simulink model "recursive_variable_window_size_alg_RL"  (R2019b)
settings: Solver=ode45  StartTime=0.0  StopTime=0.6  MaxStep=1e-4  RelTol=1e-4  AbsTol=1e-6
values from neighbouring files (symbols this model uses):
  den = [1]    [dab1.m]
  dx = 0    [dab1.m]
  num = [1]    [dab1.m]
libraries: elements x2, simulink x2, simulink_extras x1
settings Model: ExtModeTrigMode=oneshot  ExtModeArmWhenConnect=off  Creator=PC  LastModifiedBy=bae_rashid
settings SolverCC: AutoScaleAbsTol=off
settings DataIOCC: SaveFormat=Array  ReturnWorkspaceOutputs=off
settings OptimizationCC: BlockReduction=off  BooleanDataType=off  LifeSpan=inf
settings DebuggingCC: SaveWithParameterizedLinksMsg=none  UnderspecifiedInitializationDetection=Classic  MergeDetectMultiDrivingBlocksExec=none  SignalResolutionControl=TryResolveAllWithWarning  MultiTaskDSMMsg=warning  MultiTaskCondExecSysMsg=none  SFUnexpectedBacktrackingDiag=warning  SFNoUnconditionalDefaultTransitionDiag=warning  SFExecutionAtInitializationDiag=none  ArithmeticOperatorsInVariantConditions=warning
settings HardwareCC: ProdBitPerPointer=32  ProdBitPerSizeT=32  ProdBitPerPtrDiffT=32  ProdLargestAtomicFloat=None  ProdIntDivRoundTo=Undefined  ProdEndianess=Unspecified  ProdWordSize=32  ProdHWDeviceType=32-bit Generic  TargetUnknown=on
settings ModelReferenceCC: PropagateSignalLabelsOutOfModel=off
settings SFSimCC: SimUseLocalCustomCode=off  CustomCodeUndefinedFunction=UseInterfaceOnly
settings RTWCC: TemplateMakefile=grt_vc.tmf  RTWUseLocalCustomCode=off
settings CodeAppCC: StateflowObjectComments=on
settings GRTTargetCC: TargetLangStandard=C89/C90 (ANSI)  GeneratePreprocessorConditionals=Disable all  CombineOutputUpdateFcns=off  GRTInterface=on
settings ConfigComp: CovMetricSettings=dw  CovHtmlReporting=on  CovSaveCumulativeToWorkspaceVar=on  CovSaveSingleToWorkspaceVar=on  CovExternalEMLEnable=off

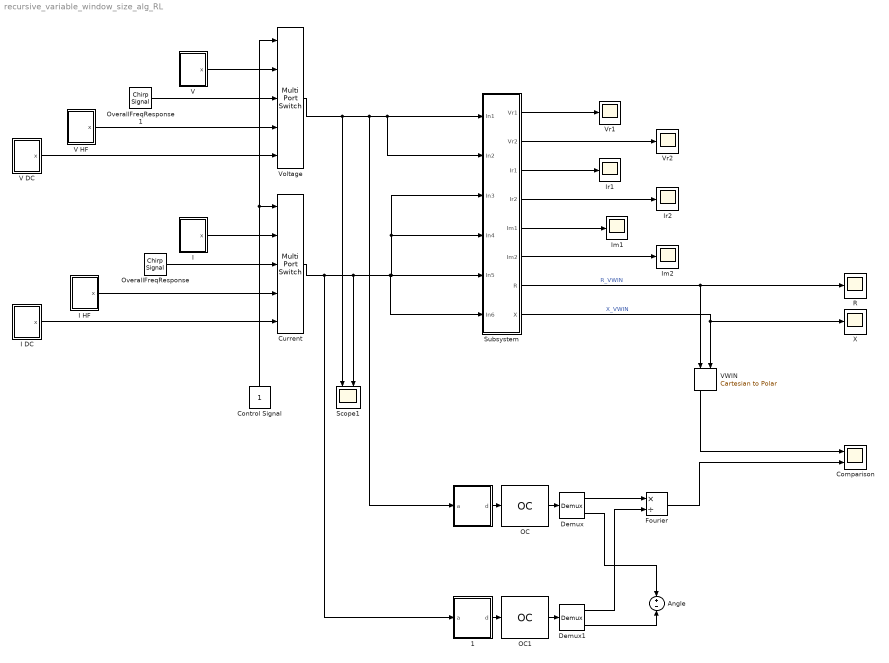
== system recursive_variable_window_size_alg_RL ==
  "  " : Subsystem  mask(Data Adquisition Board){filter=on, approx=Butterworth, order=3, numerator=[], denominator=[], freq=180, resdis=on, vertres=8, xmax=100, winsize=60, G=1.0, fs=60*60}
      mask prompts: filter "Disable Analog Filter"; approx "Filter approximation"; numerator "Free expression filter: numerator(descending order of s)"; denominator "Free expression filter: denominator:"; freq "Cut-off frequency"; resdis "Disable Vertical Resolution"; vertres "Vertical Resolution: No. of bits"; xmax "Vertical Resolution: signal range"; winsize "Window size"; G "Gain"; fs "Sampling frequency"
      mask help: Takes the instantaneous value of the input signal and convert it to the data window of samples.
      mask init:
      | dab1
      mask TypeOptions approx: Bessel | Tschebyscheff | Butterworth | free expression
      mask TypeOptions order: 2 | 3 | 4
      mask TypeOptions vertres: 8 | 12 | 16
      mask Display: disp('DAB')
  "  1" : Subsystem  mask(Data Adquisition Board){filter=on, approx=Butterworth, order=3, numerator=[], denominator=[], freq=180, resdis=on, vertres=8, xmax=100, winsize=60, G=1.0, fs=60*60}
      mask prompts: filter "Disable Analog Filter"; approx "Filter approximation"; numerator "Free expression filter: numerator(descending order of s)"; denominator "Free expression filter: denominator:"; freq "Cut-off frequency"; resdis "Disable Vertical Resolution"; vertres "Vertical Resolution: No. of bits"; xmax "Vertical Resolution: signal range"; winsize "Window size"; G "Gain"; fs "Sampling frequency"
      mask help: Takes the instantaneous value of the input signal and convert it to the data window of samples.
      mask init:
      | dab1
      mask TypeOptions approx: Bessel | Tschebyscheff | Butterworth | free expression
      mask TypeOptions order: 2 | 3 | 4
      mask TypeOptions vertres: 8 | 12 | 16
      mask Display: disp('DAB')
  Angle : Sum  Inputs=+-
  Comparison : Scope  NumInputPorts=2
  Control Signal : Constant
  Current : MultiPortSwitch  Inputs=4
  Demux : Demux  Outputs=2
  Demux1 : Demux  Outputs=2
  Fourier : Product  Inputs=*/
  I : Subsystem  mask(Signal Generator){A1=2, f1=60, A2=0, f2=2*60, A3=0, f3=5*60, tstart=1.5/60, bias=0}
      mask prompts: A1 "Amplitude 1"; f1 "Frequency 1 [Hz]"; A2 "Amplitude 2"; f2 "Frequency 2 [Hz]"; A3 "Amplitude 3"; f3 "Frequency 3 [Hz]"; tstart "Start time [sec]"
  I DC : Subsystem  mask(Signal Generator){A1=2, f1=60, A2=0, f2=2*60, A3=0, f3=3*60, tstart=1.5/60, phase1=pi/4*0, bias=0}
      mask prompts: A1 "Amplitude 1"; f1 "Frequency 1 [Hz]"; A2 "Amplitude 2"; f2 "Frequency 2 [Hz]"; A3 "Amplitude 3"; f3 "Frequency 3 [Hz]"; tstart "Start time [sec]"; phase1 "Phase 1"
  I HF : Subsystem  mask(Signal Generator){A1=2, f1=60, A2=1, f2=2*60, A3=0.3, f3=3*60, tstart=1.5/60, phase1=pi/4*0, bias=0}
      mask prompts: A1 "Amplitude 1"; f1 "Frequency 1 [Hz]"; A2 "Amplitude 2"; f2 "Frequency 2 [Hz]"; A3 "Amplitude 3"; f3 "Frequency 3 [Hz]"; tstart "Start time [sec]"; phase1 "Phase 1"
  Im1 : Scope
  Im2 : Scope
  Ir1 : Scope
  Ir2 : Scope
  OC : elements/OC  tfilt=Fourier  rfilt=[ ]  ifilt=[ ]  tlen=half  N1=60
  OC1 : elements/OC  tfilt=Fourier  rfilt=[ ]  ifilt=[ ]  tlen=full  N1=60
  OverallFreqResponse : simulink/Sources/Chirp Signal  f1=0  T=3  f2=180
  OverallFreqResponse1 : simulink/Sources/Chirp Signal  f1=0  T=3  f2=180
  R : Scope
  Scope1 : Scope  NumInputPorts=2
  Subsystem : Subsystem  mask{sr=60*60, ws_start=30, ws_end=60, t_switch=0.3}
      mask prompts: sr "Sampling Rate [Hz]"; ws_start "Initial Window Size [# of Samples]"; ws_end "Final Window Size [# of Samples]"; t_switch "Time to extend window [sec]"
  V : Subsystem  mask(Signal Generator){A1=10*sqrt(2), f1=60, A2=0, f2=2*60, A3=0, f3=5*60, tstart=1.5/60, phase1=pi/4*1, bias=0}
      mask prompts: A1 "Amplitude 1"; f1 "Frequency 1 [Hz]"; A2 "Amplitude 2"; f2 "Frequency 2 [Hz]"; A3 "Amplitude 3"; f3 "Frequency 3 [Hz]"; tstart "Start time [sec]"; phase1 "Phase 1"
  V DC : Subsystem  mask(Signal Generator){A1=10, f1=60, A2=0, f2=2*60, A3=0, f3=5*60, tstart=1.5/60, phase1=pi/4*1, bias=5}
      mask prompts: A1 "Amplitude 1"; f1 "Frequency 1 [Hz]"; A2 "Amplitude 2"; f2 "Frequency 2 [Hz]"; A3 "Amplitude 3"; f3 "Frequency 3 [Hz]"; tstart "Start time [sec]"; phase1 "Phase 1"
  V HF : Subsystem  mask(Signal Generator){A1=10, f1=60, A2=2, f2=9*60, A3=3, f3=11*60, tstart=1.5/60, phase1=pi/4*1, bias=0}
      mask prompts: A1 "Amplitude 1"; f1 "Frequency 1 [Hz]"; A2 "Amplitude 2"; f2 "Frequency 2 [Hz]"; A3 "Amplitude 3"; f3 "Frequency 3 [Hz]"; tstart "Start time [sec]"; phase1 "Phase 1"
  VWIN : simulink_extras/Transformations/Cartesian to Polar
      settings: SourceProductName=Simulink
  Voltage : MultiPortSwitch  Inputs=4
  Vr1 : Scope
  Vr2 : Scope
  X : Scope
  wires:
  Subsystem/1(Vr1) -> Vr1/1
  Subsystem/2(Vr2) -> Vr2/1
  Subsystem/3(Ir1) -> Ir1/1
  Subsystem/4(Ir2) -> Ir2/1
  Subsystem/5(Im1) -> Im1/1
  Subsystem/7(R) -> VWIN/1, R/1  "R_VWIN"
  Subsystem/8(X) -> VWIN/2, X/1  "X_VWIN"
  Subsystem/6(Im2) -> Im2/1
  Control Signal/1 -> Current/1, Voltage/1
  V/1(x) -> Voltage/2
  I/1(x) -> Current/2
  OverallFreqResponse/1 -> Current/3
  OverallFreqResponse1/1 -> Voltage/3
  V HF/1(x) -> Voltage/4
  I HF/1(x) -> Current/4
  V DC/1(x) -> Voltage/5
  I DC/1(x) -> Current/5
  "  "/1(d) -> OC/1
  Voltage/1 -> Subsystem/1(In1), Subsystem/2(In2), "  "/1(a), Scope1/1
  OC/1 -> Demux/1
  OC1/1 -> Demux1/1
  Current/1 -> "  1"/1(a), Subsystem/5(In5), Subsystem/3(In3), Subsystem/4(In4), Subsystem/6(In6), Scope1/2
  "  1"/1(d) -> OC1/1
  Demux/1 -> Fourier/1
  Demux1/1 -> Fourier/2
  Demux/2 -> Angle/1
  Demux1/2 -> Angle/2
  VWIN/1 -> Comparison/1
  Fourier/1 -> Comparison/2

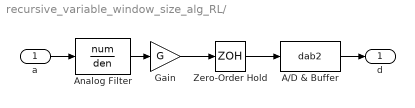
== system recursive_variable_window_size_alg_RL/   ==
  a : Inport
  A/D & Buffer : S-Function  FunctionName=dab2  Parameters=winsize,fs,dx,resdis  SFunctionDeploymentMode=off  EnableBusSupport=off
  Analog Filter : TransferFcn  Numerator=num  Denominator=den
  Gain : Gain  Gain=G  SaturateOnIntegerOverflow=on  OutDataTypeStr=Inherit: Same as input  ParamDataTypeStr=Inherit: Same as input
  Zero-Order Hold : ZeroOrderHold  SampleTime=1/fs
  d : Outport  InitialOutput=[zeros(winsize,1)]
  wires:
  Analog Filter/1 -> Gain/1
  Gain/1 -> Zero-Order Hold/1
  Zero-Order Hold/1 -> A/D & Buffer/1
  a/1 -> Analog Filter/1
  A/D & Buffer/1 -> d/1

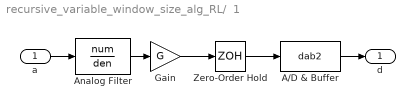
== system recursive_variable_window_size_alg_RL/  1 ==
  a : Inport
  A/D & Buffer : S-Function  FunctionName=dab2  Parameters=winsize,fs,dx,resdis  SFunctionDeploymentMode=off  EnableBusSupport=off
  Analog Filter : TransferFcn  Numerator=num  Denominator=den
  Gain : Gain  Gain=G  SaturateOnIntegerOverflow=on  OutDataTypeStr=Inherit: Same as input  ParamDataTypeStr=Inherit: Same as input
  Zero-Order Hold : ZeroOrderHold  SampleTime=1/fs
  d : Outport  InitialOutput=[zeros(winsize,1)]
  wires:
  Analog Filter/1 -> Gain/1
  Gain/1 -> Zero-Order Hold/1
  Zero-Order Hold/1 -> A/D & Buffer/1
  a/1 -> Analog Filter/1
  A/D & Buffer/1 -> d/1

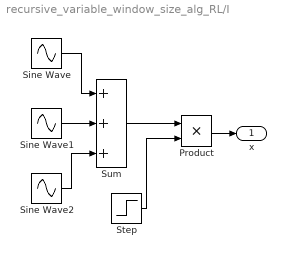
== system recursive_variable_window_size_alg_RL/I ==
  Product : Product  SaturateOnIntegerOverflow=on  RndMeth=Zero  InputSameDT=on  OutDataTypeStr=Inherit: Same as first input
  Sine Wave : Sin  Amplitude=A1  Bias=bias  Frequency=f1*2*pi  SampleTime=0
  Sine Wave1 : Sin  Amplitude=A2  Bias=bias  Frequency=f2*2*pi  SampleTime=0
  Sine Wave2 : Sin  Amplitude=A3  Bias=bias  Frequency=f3*2*pi  SampleTime=0
  Step : Step  Time=tstart
  Sum : Sum  Inputs=+++  SaturateOnIntegerOverflow=on  InputSameDT=on  OutDataTypeStr=Inherit: Same as first input
  x : Outport  InitialOutput=0
  wires:
  Sine Wave/1 -> Sum/1
  Sine Wave1/1 -> Sum/2
  Sine Wave2/1 -> Sum/3
  Sum/1 -> Product/1
  Step/1 -> Product/2
  Product/1 -> x/1

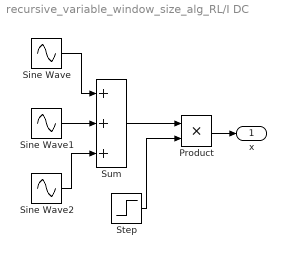
== system recursive_variable_window_size_alg_RL/I DC ==
  Product : Product  SaturateOnIntegerOverflow=on  RndMeth=Zero  InputSameDT=on  OutDataTypeStr=Inherit: Same as first input
  Sine Wave : Sin  Amplitude=A1  Bias=bias  Frequency=f1*2*pi  Phase=phase1  SampleTime=0
  Sine Wave1 : Sin  Amplitude=A2  Bias=bias  Frequency=f2*2*pi  Phase=phase1  SampleTime=0
  Sine Wave2 : Sin  Amplitude=A3  Bias=bias  Frequency=f3*2*pi  Phase=phase1  SampleTime=0
  Step : Step  Time=tstart
  Sum : Sum  Inputs=+++  SaturateOnIntegerOverflow=on  InputSameDT=on  OutDataTypeStr=Inherit: Same as first input
  x : Outport  InitialOutput=0
  wires:
  Sine Wave/1 -> Sum/1
  Sine Wave1/1 -> Sum/2
  Sine Wave2/1 -> Sum/3
  Sum/1 -> Product/1
  Step/1 -> Product/2
  Product/1 -> x/1

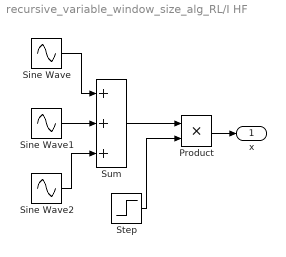
== system recursive_variable_window_size_alg_RL/I HF ==
  Product : Product  SaturateOnIntegerOverflow=on  RndMeth=Zero  InputSameDT=on  OutDataTypeStr=Inherit: Same as first input
  Sine Wave : Sin  Amplitude=A1  Frequency=f1*2*pi  Phase=phase1  SampleTime=bias
  Sine Wave1 : Sin  Amplitude=A2  Frequency=f2*2*pi  Phase=phase1  SampleTime=bias
  Sine Wave2 : Sin  Amplitude=A3  Frequency=f3*2*pi  Phase=phase1  SampleTime=bias
  Step : Step  Time=tstart
  Sum : Sum  Inputs=+++  SaturateOnIntegerOverflow=on  InputSameDT=on  OutDataTypeStr=Inherit: Same as first input
  x : Outport  InitialOutput=0
  wires:
  Sine Wave/1 -> Sum/1
  Sine Wave1/1 -> Sum/2
  Sine Wave2/1 -> Sum/3
  Sum/1 -> Product/1
  Step/1 -> Product/2
  Product/1 -> x/1

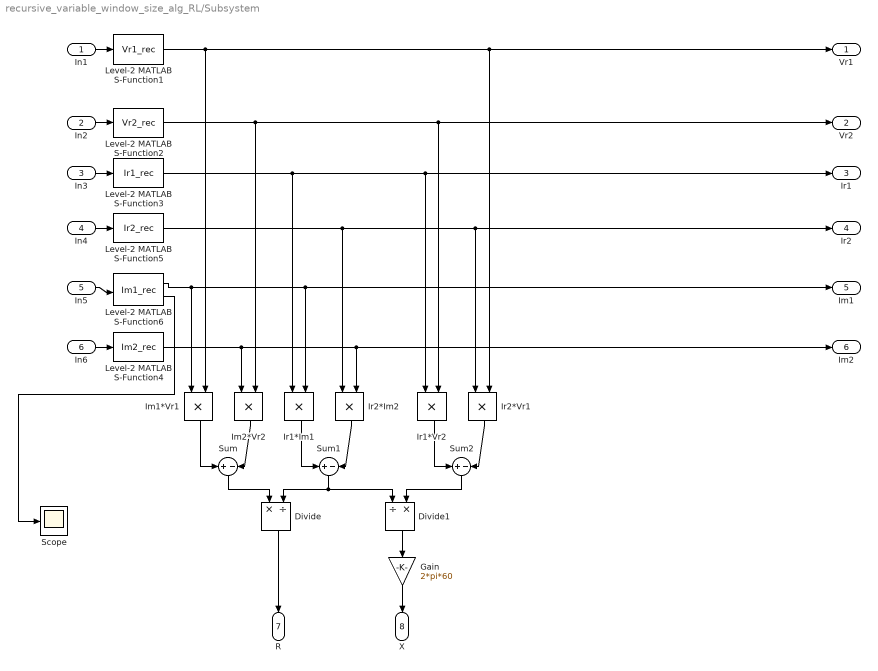
== system recursive_variable_window_size_alg_RL/Subsystem ==
  In1 : Inport
  In2 : Inport  Port=2
  In3 : Inport  Port=3
  In4 : Inport  Port=4
  In5 : Inport  Port=5
  In6 : Inport  Port=6
  Divide : Product  Inputs=*/
  Divide1 : Product  Inputs=/*
  Gain : Gain  Gain=2*pi*60
  Im1*Vr1 : Product  SaturateOnIntegerOverflow=on  RndMeth=Zero  InputSameDT=on  OutDataTypeStr=Inherit: Same as first input
  Im2*Vr2 : Product  SaturateOnIntegerOverflow=on  RndMeth=Zero  InputSameDT=on  OutDataTypeStr=Inherit: Same as first input
  Ir1*Im1 : Product  SaturateOnIntegerOverflow=on  RndMeth=Zero  InputSameDT=on  OutDataTypeStr=Inherit: Same as first input
  Ir1*Vr2 : Product  SaturateOnIntegerOverflow=on  RndMeth=Zero  InputSameDT=on  OutDataTypeStr=Inherit: Same as first input
  Ir2*Im2 : Product  SaturateOnIntegerOverflow=on  RndMeth=Zero  InputSameDT=on  OutDataTypeStr=Inherit: Same as first input
  Ir2*Vr1 : Product  SaturateOnIntegerOverflow=on  RndMeth=Zero  InputSameDT=on  OutDataTypeStr=Inherit: Same as first input
  Level-2 MATLAB S-Function1 : M-S-Function  FunctionName=Vr1_rec  Parameters=sr,ws_start,ws_end,t_switch
  Level-2 MATLAB S-Function2 : M-S-Function  FunctionName=Vr2_rec  Parameters=sr,ws_start,ws_end,t_switch
  Level-2 MATLAB S-Function3 : M-S-Function  FunctionName=Ir1_rec  Parameters=sr,ws_start,ws_end,t_switch
  Level-2 MATLAB S-Function4 : M-S-Function  FunctionName=Im2_rec  Parameters=sr,ws_start,ws_end,t_switch
  Level-2 MATLAB S-Function5 : M-S-Function  FunctionName=Ir2_rec  Parameters=sr,ws_start,ws_end,t_switch
  Level-2 MATLAB S-Function6 : M-S-Function  FunctionName=Im1_rec  Parameters=sr,ws_start,ws_end,t_switch
  Scope : Scope
  Sum : Sum  Inputs=+-
  Sum1 : Sum  Inputs=+-
  Sum2 : Sum  Inputs=+-
  Vr1 : Outport
  Vr2 : Outport  Port=2
  Ir1 : Outport  Port=3
  Ir2 : Outport  Port=4
  Im1 : Outport  Port=5
  Im2 : Outport  Port=6
  R : Outport  Port=7
  X : Outport  Port=8
  wires:
  In2/1 -> Level-2 MATLAB S-Function2/1
  Level-2 MATLAB S-Function4/1 -> Im2*Vr2/1, Ir2*Im2/2, Im2/1
  In1/1 -> Level-2 MATLAB S-Function1/1
  In5/1 -> Level-2 MATLAB S-Function6/1
  Level-2 MATLAB S-Function6/1 -> Ir1*Im1/2, Im1/1, Im1*Vr1/1
  Level-2 MATLAB S-Function3/1 -> Ir1*Im1/1, Ir1*Vr2/1, Ir1/1
  In3/1 -> Level-2 MATLAB S-Function3/1
  Level-2 MATLAB S-Function1/1 -> Ir2*Vr1/2, Vr1/1, Im1*Vr1/2
  In4/1 -> Level-2 MATLAB S-Function5/1
  Level-2 MATLAB S-Function5/1 -> Ir2*Im2/1, Ir2*Vr1/1, Ir2/1
  In6/1 -> Level-2 MATLAB S-Function4/1
  Level-2 MATLAB S-Function2/1 -> Im2*Vr2/2, Ir1*Vr2/2, Vr2/1
  Im1*Vr1/1 -> Sum/1
  Im2*Vr2/1 -> Sum/2
  Ir1*Im1/1 -> Sum1/1
  Ir2*Im2/1 -> Sum1/2
  Sum/1 -> Divide/1
  Sum1/1 -> Divide/2, Divide1/1
  Divide/1 -> R/1
  Ir1*Vr2/1 -> Sum2/1
  Ir2*Vr1/1 -> Sum2/2
  Sum2/1 -> Divide1/2
  Divide1/1 -> Gain/1
  Gain/1 -> X/1
  Level-2 MATLAB S-Function6/2 -> Scope/1

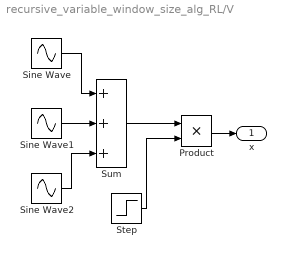
== system recursive_variable_window_size_alg_RL/V ==
  Product : Product  SaturateOnIntegerOverflow=on  RndMeth=Zero  InputSameDT=on  OutDataTypeStr=Inherit: Same as first input
  Sine Wave : Sin  Amplitude=A1  Bias=bias  Frequency=f1*2*pi  Phase=phase1  SampleTime=0
  Sine Wave1 : Sin  Amplitude=A2  Bias=bias  Frequency=f2*2*pi  Phase=phase1  SampleTime=0
  Sine Wave2 : Sin  Amplitude=A3  Bias=bias  Frequency=f3*2*pi  Phase=phase1  SampleTime=0
  Step : Step  Time=tstart
  Sum : Sum  Inputs=+++  SaturateOnIntegerOverflow=on  InputSameDT=on  OutDataTypeStr=Inherit: Same as first input
  x : Outport  InitialOutput=0
  wires:
  Sine Wave/1 -> Sum/1
  Sine Wave1/1 -> Sum/2
  Sine Wave2/1 -> Sum/3
  Sum/1 -> Product/1
  Step/1 -> Product/2
  Product/1 -> x/1

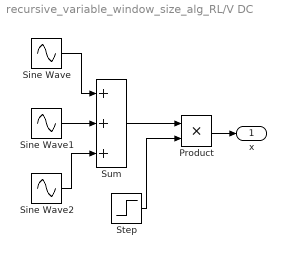
== system recursive_variable_window_size_alg_RL/V DC ==
  Product : Product  SaturateOnIntegerOverflow=on  RndMeth=Zero  InputSameDT=on  OutDataTypeStr=Inherit: Same as first input
  Sine Wave : Sin  Amplitude=A1  Bias=bias  Frequency=f1*2*pi  Phase=phase1  SampleTime=0
  Sine Wave1 : Sin  Amplitude=A2  Bias=bias  Frequency=f2*2*pi  Phase=phase1  SampleTime=0
  Sine Wave2 : Sin  Amplitude=A3  Bias=bias  Frequency=f3*2*pi  Phase=phase1  SampleTime=0
  Step : Step  Time=tstart
  Sum : Sum  Inputs=+++  SaturateOnIntegerOverflow=on  InputSameDT=on  OutDataTypeStr=Inherit: Same as first input
  x : Outport  InitialOutput=0
  wires:
  Sine Wave/1 -> Sum/1
  Sine Wave1/1 -> Sum/2
  Sine Wave2/1 -> Sum/3
  Sum/1 -> Product/1
  Step/1 -> Product/2
  Product/1 -> x/1

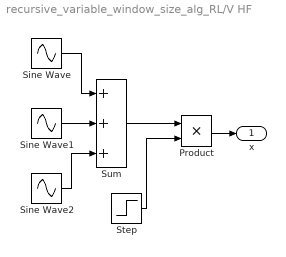
== system recursive_variable_window_size_alg_RL/V HF ==
  Product : Product  SaturateOnIntegerOverflow=on  RndMeth=Zero  InputSameDT=on  OutDataTypeStr=Inherit: Same as first input
  Sine Wave : Sin  Amplitude=A1  Bias=bias  Frequency=f1*2*pi  Phase=phase1  SampleTime=0
  Sine Wave1 : Sin  Amplitude=A2  Bias=bias  Frequency=f2*2*pi  Phase=phase1  SampleTime=0
  Sine Wave2 : Sin  Amplitude=A3  Bias=bias  Frequency=f3*2*pi  Phase=phase1  SampleTime=0
  Step : Step  Time=tstart
  Sum : Sum  Inputs=+++  SaturateOnIntegerOverflow=on  InputSameDT=on  OutDataTypeStr=Inherit: Same as first input
  x : Outport  InitialOutput=0
  wires:
  Sine Wave/1 -> Sum/1
  Sine Wave1/1 -> Sum/2
  Sine Wave2/1 -> Sum/3
  Sum/1 -> Product/1
  Step/1 -> Product/2
  Product/1 -> x/1
